simulink model "ADCS_orbiter_detumbling"  (R2022a)
settings: Solver=ode4  StartTime=0.0  StopTime=21085  FixedStep=0.1  MaxStep=1  RelTol=1e-8
values from neighbouring files (symbols this model uses):
  A_cube = 1    [Data_detumbling.m]    (also in main_orbiter_detumbling.m = 12.9)
  A_S2B = [1,0,0;0,-1,0;0,0,-1]    [Data_detumbling.m]
  alpha_x = deg2rad(6/3600)    [Data_detumbling.m]
  alpha_y = deg2rad(6/3600)    [Data_detumbling.m]
  alpha_z = deg2rad(40/3600)    [Data_detumbling.m]
  B_ast = pinv(B)    [Data_detumbling.m]
  ceps = cos(eps)    [Data_detumbling.m]    (also in main_orbiter_detumbling.m)
  F_max = 0.650    (= 0.65)    [Data_detumbling.m]    (also in main_orbiter_detumbling.m = 1.13)
  F_min = 0.160    (= 0.16)    [Data_detumbling.m]    (also in main_orbiter_detumbling.m = 0.19)
  J = [Jx,0,0 ... (first row only)    [Data_detumbling.m]    (also in DisturbanceEvaluation.m = {J_NSO; J_SO}; Thruster_sizing_2.m = diag([12043.36, 15990.19, 8547.84]); main_orbiter.m = J_SO; main_orbiter_detumbling.m = J_SO)
  k_dx = G*J(1,1)/max(diag(J))    [main_orbiter_detumbling.m]
  k_dy = G*J(2,2)/max(diag(J))    [main_orbiter_detumbling.m]
  k_dz = G*J(3,3)/max(diag(J))    [main_orbiter_detumbling.m]
  k_p = 0    [Data_detumbling.m]    (also in main_orbiter_detumbling.m)
  n1 = [1;0;0]    [Data_detumbling.m]    (also in main_orbiter_detumbling.m)
  n2 = [0;1;0]    [Data_detumbling.m]    (also in main_orbiter_detumbling.m)
  n3 = [0;0;1]    [Data_detumbling.m]    (also in main_orbiter_detumbling.m)
  n4 = -n1    [Data_detumbling.m]    (also in main_orbiter_detumbling.m)
  n5 = -n2    [Data_detumbling.m]    (also in main_orbiter_detumbling.m)
  n6 = -n3    [Data_detumbling.m]    (also in main_orbiter_detumbling.m)
  n_sun = 2*pi/(365.25*24*3600)    (= 1.99102127766e-07)    [Data_detumbling.m]    (also in main_orbiter_detumbling.m)
  P = F_e/c    [Data_detumbling.m]    (also in main_orbiter_detumbling.m)
  qbn0 = qrand./norm(qrand)    [main_orbiter.m]    (also in main_orbiter_detumbling.m)
  R = diag([lx_mb/2 ly_mb/2 lz_mb/2]) * [0  0  1  1  0  0 -1 -1 ... (first row only)    [Data_detumbling.m]    (also in main_orbiter_detumbling.m = 0.5*[-ly*cos(inc)              ly*cos(inc)            ly*cos)
  R_ast = pinv(R)    [Data_detumbling.m]    (also in main_orbiter_detumbling.m)
  r_i = r_cube * [n1,n2,n3,n4,n5,n6]    [Data_detumbling.m]    (also in main_orbiter_detumbling.m = [lx/2-cm_off_x  -cm_off_x       -cm_off_x        lx/2+cm_off)
  rho_d = 0.1    [Data_detumbling.m]    (also in main_orbiter_detumbling.m)
  rho_s = 0.5    [Data_detumbling.m]    (also in main_orbiter_detumbling.m)
  S_star1 = S_star1/norm(S_star1)    [Data_detumbling.m]
  S_star2 = S_star2/norm(S_star2)    [Data_detumbling.m]
  S_star3 = S_star3/norm(S_star3)    [Data_detumbling.m]
  S_star4 = S_star4/norm(S_star4)    [Data_detumbling.m]
  seps = sin(eps)    [Data_detumbling.m]    (also in main_orbiter_detumbling.m)
  sigma_ARW = deg2rad(0.001)    [main_orbiter_detumbling.m]
  state0 = [r_vec_new; v_vec_new]    [main_orbiter_detumbling.m]
  w = ones(length(R(1,:)),1)    [Data_detumbling.m]    (also in main_orbiter_detumbling.m)
  w_c = [0 0 0]'    [Data_detumbling.m]    (also in main_orbiter_detumbling.m)
  wb0 = 0.0001*rand(3, 1)    [main_orbiter.m]    (also in main_orbiter_detumbling.m = 0.1*rand(3, 1))
libraries: vrlib x8, matrix_library x1, simulink x1
(part 2 of 3)

== system ADCS_orbiter_detumbling/Actuators/Subsystem4/If Action Subsystem ==
  In1 : Inport
  Action Port : ActionPort  ActionPortLabel=if(u1 > F_max)
  Out1 : Outport
  wires:
  In1/1 -> Out1/1

== system ADCS_orbiter_detumbling/Actuators/Subsystem4/If Action Subsystem1 ==
  In1 : Inport
  Action Port : ActionPort  ActionPortLabel=elseif(u1<F_min)
  Out1 : Outport
  wires:
  In1/1 -> Out1/1

== system ADCS_orbiter_detumbling/Actuators/Subsystem4/If Action Subsystem2 ==
  In1 : Inport
  Action Port : ActionPort  ActionPortLabel=else
  Out1 : Outport
  wires:
  In1/1 -> Out1/1

== system ADCS_orbiter_detumbling/Actuators/Subsystem5/If Action Subsystem ==
  In1 : Inport
  Action Port : ActionPort  ActionPortLabel=if(u1 > F_max)
  Out1 : Outport
  wires:
  In1/1 -> Out1/1

== system ADCS_orbiter_detumbling/Actuators/Subsystem5/If Action Subsystem1 ==
  In1 : Inport
  Action Port : ActionPort  ActionPortLabel=elseif(u1<F_min)
  Out1 : Outport
  wires:
  In1/1 -> Out1/1

== system ADCS_orbiter_detumbling/Actuators/Subsystem5/If Action Subsystem2 ==
  In1 : Inport
  Action Port : ActionPort  ActionPortLabel=else
  Out1 : Outport
  wires:
  In1/1 -> Out1/1

== system ADCS_orbiter_detumbling/Actuators/Subsystem6/If Action Subsystem ==
  In1 : Inport
  Action Port : ActionPort  ActionPortLabel=if(u1 > F_max)
  Out1 : Outport
  wires:
  In1/1 -> Out1/1

== system ADCS_orbiter_detumbling/Actuators/Subsystem6/If Action Subsystem1 ==
  In1 : Inport
  Action Port : ActionPort  ActionPortLabel=elseif(u1<F_min)
  Out1 : Outport
  wires:
  In1/1 -> Out1/1

== system ADCS_orbiter_detumbling/Actuators/Subsystem6/If Action Subsystem2 ==
  In1 : Inport
  Action Port : ActionPort  ActionPortLabel=else
  Out1 : Outport
  wires:
  In1/1 -> Out1/1

== system ADCS_orbiter_detumbling/Actuators/Subsystem7/If Action Subsystem ==
  In1 : Inport
  Action Port : ActionPort  ActionPortLabel=if(u1 > F_max)
  Out1 : Outport
  wires:
  In1/1 -> Out1/1

== system ADCS_orbiter_detumbling/Actuators/Subsystem7/If Action Subsystem1 ==
  In1 : Inport
  Action Port : ActionPort  ActionPortLabel=elseif(u1<F_min)
  Out1 : Outport
  wires:
  In1/1 -> Out1/1

== system ADCS_orbiter_detumbling/Actuators/Subsystem7/If Action Subsystem2 ==
  In1 : Inport
  Action Port : ActionPort  ActionPortLabel=else
  Out1 : Outport
  wires:
  In1/1 -> Out1/1

== system ADCS_orbiter_detumbling/Actuators/Subsystem8/If Action Subsystem ==
  In1 : Inport
  Action Port : ActionPort  ActionPortLabel=if(u1 > 0)
  Out2 : Outport
  wires:
  In1/1 -> Out2/1

== system ADCS_orbiter_detumbling/Actuators/Subsystem8/If Action Subsystem1 ==
  In1 : Inport
  Input : Inport  Port=2
  Input1 : Inport  Port=3
  Action Port : ActionPort  ActionPortLabel=else
  If : If  NumInputs=2  IfExpression=u1 > 0 & u2==0
  If Action Subsystem : Subsystem  TreatAsAtomicUnit=on
  If Action Subsystem1 : Subsystem  TreatAsAtomicUnit=on
  Merge : Merge
  Out1 : Outport
  wires:
  In1/1 -> If Action Subsystem1/1(In1)
  Input/1 -> If/1  "u(k-1)"
  Input1/1 -> If/2  "u(k-2)"
  If/1 -> If Action Subsystem/Action
  If/2 -> If Action Subsystem1/Action
  If Action Subsystem1/1(Out1) -> Merge/2
  If Action Subsystem/1(Out1) -> Merge/1
  Merge/1 -> Out1/1

== system ADCS_orbiter_detumbling/Actuators/Subsystem9/If Action Subsystem ==
  In1 : Inport
  Action Port : ActionPort  ActionPortLabel=if(u1 > 0)
  Out2 : Outport
  wires:
  In1/1 -> Out2/1

== system ADCS_orbiter_detumbling/Actuators/Subsystem9/If Action Subsystem1 ==
  In1 : Inport
  Input : Inport  Port=2
  Input1 : Inport  Port=3
  Action Port : ActionPort  ActionPortLabel=else
  If : If  NumInputs=2  IfExpression=u1 > 0 & u2==0
  If Action Subsystem : Subsystem  TreatAsAtomicUnit=on
  If Action Subsystem1 : Subsystem  TreatAsAtomicUnit=on
  Merge : Merge
  Out1 : Outport
  wires:
  Merge/1 -> Out1/1
  If Action Subsystem/1(Out1) -> Merge/1
  If Action Subsystem1/1(Out1) -> Merge/2
  If/2 -> If Action Subsystem1/Action
  If/1 -> If Action Subsystem/Action
  Input1/1 -> If/2  "u(k-2)"
  Input/1 -> If/1  "u(k-1)"
  In1/1 -> If Action Subsystem1/1(In1)

== system ADCS_orbiter_detumbling/Control/target quaterion/Mapping choice ==
  A_I2B_target : Inport
  From q4 : Subsystem
  If Action Subsystem2 : Subsystem  TreatAsAtomicUnit=on
  If Action Subsystem3 : Subsystem  TreatAsAtomicUnit=on
  If1 : If  NumInputs=2  IfExpression=u1 == u2
  Max : MinMax  Function=max  Inputs=4
  Merge1 : Merge
  q_1 : Subsystem
  q_2 : Subsystem
  q_3 : Subsystem
  q_4 : Subsystem
  q_c : Outport
  wires:
  Merge1/1 -> q_c/1  "q_err"
  q_4/1(q4) -> Max/4, From q4/2(q4), If1/1  "q4"
  q_3/1(q3) -> Max/3, If Action Subsystem2/5(q3)  "q3"
  q_2/1(q2) -> Max/2, If Action Subsystem2/4(q2)  "q2"
  q_1/1(q1) -> Max/1, If Action Subsystem2/3(q1)  "q1"
  Max/1 -> If1/2, If Action Subsystem2/1(max)  "max"
  From q4/1(q_err) -> If Action Subsystem3/1(q_err)
  If Action Subsystem3/1("q_err from q4 ") -> Merge1/1
  A_I2B_target/1 -> If Action Subsystem2/2(A_I2B_err), q_1/1(A_I2B_err), q_2/1(A_I2B_err), From q4/1(A_I2B_err), q_4/1(A_I2B_err), q_3/1(A_I2B_err)
  If1/1 -> If Action Subsystem3/Action
  If1/2 -> If Action Subsystem2/Action
  If Action Subsystem2/1(Output) -> Merge1/2

== system ADCS_orbiter_detumbling/Environment 2/ShadowCylinder/If Action Subsystem ==
  Action Port : ActionPort  ActionPortLabel=if(u1 > 0)
  Constant : Constant
  Out1 : Outport
  wires:
  Constant/1 -> Out1/1

== system ADCS_orbiter_detumbling/Environment 2/ShadowCylinder/If Action Subsystem1 ==
  In1 : Inport
  Action Port : ActionPort  ActionPortLabel=else
  If : If
  If Action Subsystem : Subsystem  TreatAsAtomicUnit=on
  If Action Subsystem1 : Subsystem  TreatAsAtomicUnit=on
  Merge : Merge
  Out1 : Outport
  wires:
  In1/1 -> If/1
  If/1 -> If Action Subsystem/Action
  Merge/1 -> Out1/1
  If Action Subsystem/1(Out1) -> Merge/1
  If Action Subsystem1/1(Out1) -> Merge/2
  If/2 -> If Action Subsystem1/Action

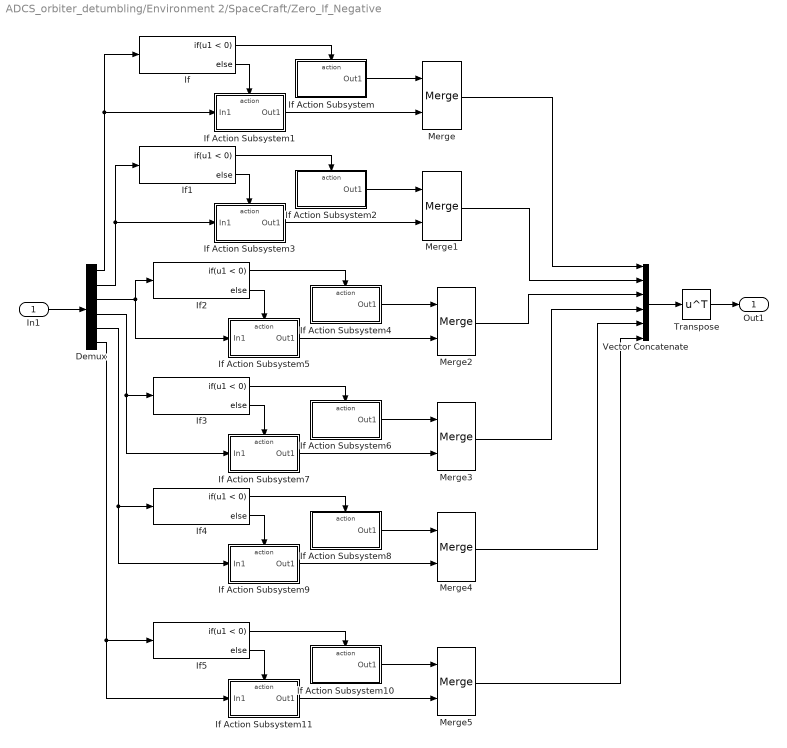
== system ADCS_orbiter_detumbling/Environment 2/SpaceCraft/Zero_If_Negative ==
  In1 : Inport
  Demux : Demux  Outputs=6
  If{,1..5} (6 alike) : If  IfExpression=u1 < 0
  If Action Subsystem : Subsystem  TreatAsAtomicUnit=on
  If Action Subsystem1 : Subsystem  TreatAsAtomicUnit=on
  If Action Subsystem10 : Subsystem  TreatAsAtomicUnit=on
  If Action Subsystem11 : Subsystem  TreatAsAtomicUnit=on
  If Action Subsystem2 : Subsystem  TreatAsAtomicUnit=on
  If Action Subsystem3 : Subsystem  TreatAsAtomicUnit=on
  If Action Subsystem4 : Subsystem  TreatAsAtomicUnit=on
  If Action Subsystem5 : Subsystem  TreatAsAtomicUnit=on
  If Action Subsystem6 : Subsystem  TreatAsAtomicUnit=on
  If Action Subsystem7 : Subsystem  TreatAsAtomicUnit=on
  If Action Subsystem8 : Subsystem  TreatAsAtomicUnit=on
  If Action Subsystem9 : Subsystem  TreatAsAtomicUnit=on
  Merge{,1..5} (6 alike) : Merge
  Transpose : Math  Operator=transpose
  Vector Concatenate : Concatenate  NumInputs=6
  Out1 : Outport
  wires:
  In1/1 -> Demux/1
  Vector Concatenate/1 -> Transpose/1
  Demux/1 -> If Action Subsystem1/1(In1), If/1
  If/1 -> If Action Subsystem/Action
  If Action Subsystem/1(Out1) -> Merge/1
  If Action Subsystem1/1(Out1) -> Merge/2
  If/2 -> If Action Subsystem1/Action
  If Action Subsystem2/1(Out1) -> Merge1/1
  Demux/2 -> If Action Subsystem3/1(In1), If1/1
  If1/1 -> If Action Subsystem2/Action
  If1/2 -> If Action Subsystem3/Action
  If Action Subsystem3/1(Out1) -> Merge1/2
  Merge/1 -> Vector Concatenate/1
  Merge1/1 -> Vector Concatenate/2
  If Action Subsystem4/1(Out1) -> Merge2/1
  Demux/3 -> If Action Subsystem5/1(In1), If2/1
  If2/1 -> If Action Subsystem4/Action
  If2/2 -> If Action Subsystem5/Action
  If Action Subsystem5/1(Out1) -> Merge2/2
  Merge2/1 -> Vector Concatenate/3
  If Action Subsystem6/1(Out1) -> Merge3/1
  Demux/4 -> If Action Subsystem7/1(In1), If3/1
  If3/1 -> If Action Subsystem6/Action
  If3/2 -> If Action Subsystem7/Action
  If Action Subsystem7/1(Out1) -> Merge3/2
  Merge3/1 -> Vector Concatenate/4
  If Action Subsystem8/1(Out1) -> Merge4/1
  Demux/5 -> If Action Subsystem9/1(In1), If4/1
  If4/1 -> If Action Subsystem8/Action
  If4/2 -> If Action Subsystem9/Action
  If Action Subsystem9/1(Out1) -> Merge4/2
  Merge4/1 -> Vector Concatenate/5
  If Action Subsystem10/1(Out1) -> Merge5/1
  Demux/6 -> If Action Subsystem11/1(In1), If5/1
  If5/1 -> If Action Subsystem10/Action
  If5/2 -> If Action Subsystem11/Action
  If Action Subsystem11/1(Out1) -> Merge5/2
  Merge5/1 -> Vector Concatenate/6
  Transpose/1 -> Out1/1

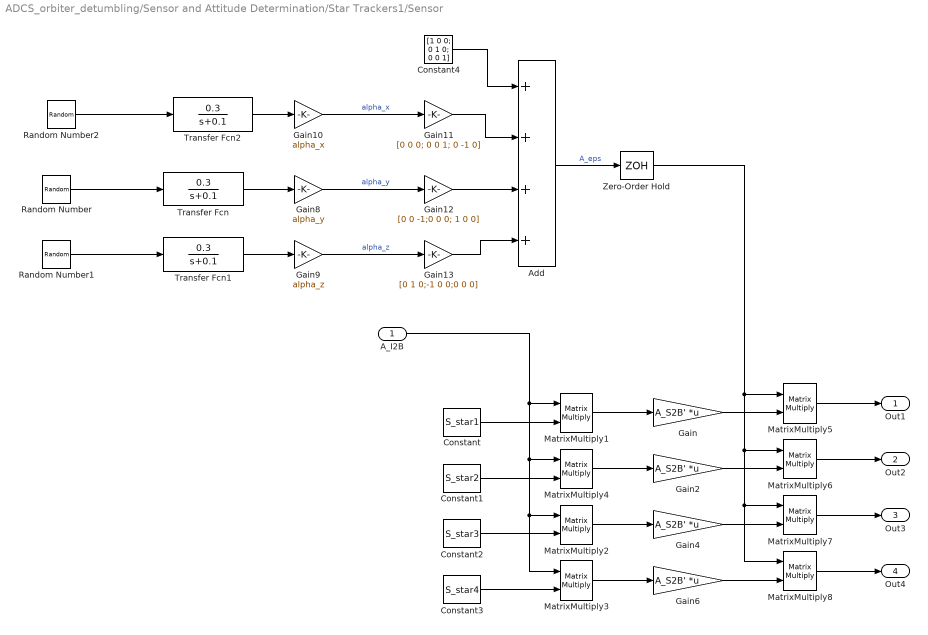
== system ADCS_orbiter_detumbling/Sensor and Attitude Determination/Star Trackers1/Sensor ==
  A_I2B : Inport
  Add : Sum  Inputs=++++
  Constant : Constant  Value=S_star1
  Constant1 : Constant  Value=S_star2
  Constant2 : Constant  Value=S_star3
  Constant3 : Constant  Value=S_star4
  Constant4 : Constant  Value=[1 0 0; 0 1 0; 0 0 1]
  Gain{,2,4,6} (4 alike) : Gain  Gain=A_S2B'  Multiplication=Matrix(K*u)
  Gain10 : Gain  Gain=alpha_x
  Gain11 : Gain  Gain=[0 0 0; 0 0 1; 0 -1 0]
  Gain12 : Gain  Gain=[0 0 -1;0 0 0; 1 0 0]
  Gain13 : Gain  Gain=[0 1 0;-1 0 0;0 0 0]
  Gain8 : Gain  Gain=alpha_y
  Gain9 : Gain  Gain=alpha_z
  MatrixMultiply{1..8} (8 alike) : Product  Multiplication=Matrix(*)
  Random Number : RandomNumber  SampleTime=0.1
  Random Number1 : RandomNumber  SampleTime=0.1
  Random Number2 : RandomNumber  SampleTime=0.1
  Transfer Fcn : TransferFcn  Numerator=[0.3]  Denominator=[1 0.1]
  Transfer Fcn1 : TransferFcn  Numerator=[0.3]  Denominator=[1 0.1]
  Transfer Fcn2 : TransferFcn  Numerator=[0.3]  Denominator=[1 0.1]
  Zero-Order Hold : ZeroOrderHold  SampleTime=-1
  Out1 : Outport
  Out2 : Outport  Port=2
  Out3 : Outport  Port=3
  Out4 : Outport  Port=4
  wires:
  MatrixMultiply1/1 -> Gain/1
  Constant/1 -> MatrixMultiply1/2
  A_I2B/1 -> MatrixMultiply3/1, MatrixMultiply2/1, MatrixMultiply4/1, MatrixMultiply1/1
  Constant1/1 -> MatrixMultiply4/2
  Gain6/1 -> MatrixMultiply8/2
  MatrixMultiply8/1 -> Out4/1
  Gain4/1 -> MatrixMultiply7/2
  MatrixMultiply6/1 -> Out2/1
  Constant3/1 -> MatrixMultiply3/2
  MatrixMultiply4/1 -> Gain2/1
  Constant2/1 -> MatrixMultiply2/2
  MatrixMultiply2/1 -> Gain4/1
  Gain2/1 -> MatrixMultiply6/2
  MatrixMultiply3/1 -> Gain6/1
  MatrixMultiply7/1 -> Out3/1
  MatrixMultiply5/1 -> Out1/1
  Gain9/1 -> Gain13/1  "alpha_z"
  Gain10/1 -> Gain11/1  "alpha_x"
  Transfer Fcn2/1 -> Gain10/1
  Random Number1/1 -> Transfer Fcn1/1
  Transfer Fcn1/1 -> Gain9/1
  Gain8/1 -> Gain12/1  "alpha_y"
  Random Number/1 -> Transfer Fcn/1
  Transfer Fcn/1 -> Gain8/1
  Random Number2/1 -> Transfer Fcn2/1
  Gain13/1 -> Add/4
  Gain12/1 -> Add/3
  Gain11/1 -> Add/2
  Constant4/1 -> Add/1
  Add/1 -> Zero-Order Hold/1  "A_eps"
  Gain/1 -> MatrixMultiply5/2
  Zero-Order Hold/1 -> MatrixMultiply5/1, MatrixMultiply6/1, MatrixMultiply7/1, MatrixMultiply8/1

== system ADCS_orbiter_detumbling/Sensor and Attitude Determination/Subsystem3/From q4 ==
  q4 : Inport
  A_I2B_err : Inport  Port=2
  Divide : Product  Inputs=*/
  Gain9 : Gain  Gain=4
  Selector3 : Selector  NumberOfDimensions=2  InputPortWidth=3  IndexOptions=Index vector (dialog),Index vector (dialog)  Indices=2,3  OutputSizes=1,1
  Selector4 : Selector  NumberOfDimensions=2  InputPortWidth=3  IndexOptions=Index vector (dialog),Index vector (dialog)  Indices=3,2  OutputSizes=1,1
  Selector5 : Selector  NumberOfDimensions=2  InputPortWidth=3  IndexOptions=Index vector (dialog),Index vector (dialog)  Indices=3,1  OutputSizes=1,1
  Selector6 : Selector  NumberOfDimensions=2  InputPortWidth=3  IndexOptions=Index vector (dialog),Index vector (dialog)  Indices=1,3  OutputSizes=1,1
  Selector7 : Selector  NumberOfDimensions=2  InputPortWidth=3  IndexOptions=Index vector (dialog),Index vector (dialog)  Indices=1,2  OutputSizes=1,1
  Selector8 : Selector  NumberOfDimensions=2  InputPortWidth=3  IndexOptions=Index vector (dialog),Index vector (dialog)  Indices=2,1  OutputSizes=1,1
  Sum1 : Sum  Inputs=+-
  Sum2 : Sum  Inputs=+-
  Sum3 : Sum  Inputs=+-
  Vector Concatenate : Concatenate
  Vector Concatenate2 : Concatenate  NumInputs=3
  q_err : Outport
  wires:
  Vector Concatenate2/1 -> Divide/1
  Selector7/1 -> Sum3/1
  Selector5/1 -> Sum2/1
  Divide/1 -> Vector Concatenate/1
  Selector3/1 -> Sum1/1
  Selector8/1 -> Sum3/2
  Sum2/1 -> Vector Concatenate2/2
  Vector Concatenate/1 -> q_err/1
  A_I2B_err/1 -> Selector3/1, Selector4/1, Selector5/1, Selector6/1, Selector7/1, Selector8/1
  Gain9/1 -> Divide/2
  Sum1/1 -> Vector Concatenate2/1
  q4/1 -> Gain9/1, Vector Concatenate/2  "q4"
  Selector4/1 -> Sum1/2
  Sum3/1 -> Vector Concatenate2/3
  Selector6/1 -> Sum2/2

== system ADCS_orbiter_detumbling/Sensor and Attitude Determination/Subsystem3/Mapping choice ==
  A_I2B_err1 : Inport
  From q4 : Subsystem
  If Action Subsystem2 : Subsystem  TreatAsAtomicUnit=on
  If Action Subsystem3 : Subsystem  TreatAsAtomicUnit=on
  If1 : If  NumInputs=2  IfExpression=u1 == u2
  Max : MinMax  Function=max  Inputs=4
  Merge1 : Merge
  q_1 : Subsystem
  q_2 : Subsystem
  q_3 : Subsystem
  q_4 : Subsystem
  q_err : Outport
  wires:
  Merge1/1 -> q_err/1  "q_err"
  q_4/1(q4) -> Max/4, From q4/2(q4), If1/1  "q4"
  q_3/1(q3) -> Max/3, If Action Subsystem2/5(q3)  "q3"
  q_2/1(q2) -> Max/2, If Action Subsystem2/4(q2)  "q2"
  q_1/1(q1) -> Max/1, If Action Subsystem2/3(q1)  "q1"
  Max/1 -> If1/2, If Action Subsystem2/1(max)  "max"
  From q4/1(q_err) -> If Action Subsystem3/1(q_err)
  If Action Subsystem3/1("q_err from q4 ") -> Merge1/1
  A_I2B_err1/1 -> If Action Subsystem2/2(A_I2B_err), q_1/1(A_I2B_err), q_2/1(A_I2B_err), From q4/1(A_I2B_err), q_4/1(A_I2B_err), q_3/1(A_I2B_err)
  If1/1 -> If Action Subsystem3/Action
  If1/2 -> If Action Subsystem2/Action
  If Action Subsystem2/1(Output) -> Merge1/2

== system ADCS_orbiter_detumbling/Actuators/Subsystem10/If Action Subsystem1/If Action Subsystem ==
  Action Port : ActionPort  ActionPortLabel=if(u1 > 0 & u2==0)
  Constant : Constant  Value=F_min
  Out1 : Outport
  wires:
  Constant/1 -> Out1/1

== system ADCS_orbiter_detumbling/Actuators/Subsystem10/If Action Subsystem1/If Action Subsystem1 ==
  In1 : Inport
  Action Port : ActionPort  ActionPortLabel=else
  Out1 : Outport
  wires:
  In1/1 -> Out1/1

== system ADCS_orbiter_detumbling/Actuators/Subsystem11/If Action Subsystem1/If Action Subsystem ==
  Action Port : ActionPort  ActionPortLabel=if(u1 > 0 & u2==0)
  Constant : Constant  Value=F_min
  Out1 : Outport
  wires:
  Constant/1 -> Out1/1

== system ADCS_orbiter_detumbling/Actuators/Subsystem11/If Action Subsystem1/If Action Subsystem1 ==
  In1 : Inport
  Action Port : ActionPort  ActionPortLabel=else
  Out1 : Outport
  wires:
  In1/1 -> Out1/1

== system ADCS_orbiter_detumbling/Actuators/Subsystem12/If Action Subsystem1/If Action Subsystem ==
  Action Port : ActionPort  ActionPortLabel=if(u1 > 0 & u2==0)
  Constant : Constant  Value=F_min
  Out1 : Outport
  wires:
  Constant/1 -> Out1/1

== system ADCS_orbiter_detumbling/Actuators/Subsystem12/If Action Subsystem1/If Action Subsystem1 ==
  In1 : Inport
  Action Port : ActionPort  ActionPortLabel=else
  Out1 : Outport
  wires:
  In1/1 -> Out1/1

== system ADCS_orbiter_detumbling/Actuators/Subsystem13/If Action Subsystem1/If Action Subsystem ==
  Action Port : ActionPort  ActionPortLabel=if(u1 > 0 & u2==0)
  Constant : Constant  Value=F_min
  Out1 : Outport
  wires:
  Constant/1 -> Out1/1

== system ADCS_orbiter_detumbling/Actuators/Subsystem13/If Action Subsystem1/If Action Subsystem1 ==
  In1 : Inport
  Action Port : ActionPort  ActionPortLabel=else
  Out1 : Outport
  wires:
  In1/1 -> Out1/1

== system ADCS_orbiter_detumbling/Actuators/Subsystem14/If Action Subsystem1/If Action Subsystem ==
  Action Port : ActionPort  ActionPortLabel=if(u1 > 0 & u2==0)
  Constant : Constant  Value=F_min
  Out1 : Outport
  wires:
  Constant/1 -> Out1/1

== system ADCS_orbiter_detumbling/Actuators/Subsystem14/If Action Subsystem1/If Action Subsystem1 ==
  In1 : Inport
  Action Port : ActionPort  ActionPortLabel=else
  Out1 : Outport
  wires:
  In1/1 -> Out1/1

== system ADCS_orbiter_detumbling/Actuators/Subsystem15/If Action Subsystem1/If Action Subsystem ==
  Action Port : ActionPort  ActionPortLabel=if(u1 > 0 & u2==0)
  Constant : Constant  Value=F_min
  Out1 : Outport
  wires:
  Constant/1 -> Out1/1

== system ADCS_orbiter_detumbling/Actuators/Subsystem15/If Action Subsystem1/If Action Subsystem1 ==
  In1 : Inport
  Action Port : ActionPort  ActionPortLabel=else
  Out1 : Outport
  wires:
  In1/1 -> Out1/1

== system ADCS_orbiter_detumbling/Actuators/Subsystem8/If Action Subsystem1/If Action Subsystem ==
  Action Port : ActionPort  ActionPortLabel=if(u1 > 0 & u2==0)
  Constant : Constant  Value=F_min
  Out1 : Outport
  wires:
  Constant/1 -> Out1/1

== system ADCS_orbiter_detumbling/Actuators/Subsystem8/If Action Subsystem1/If Action Subsystem1 ==
  In1 : Inport
  Action Port : ActionPort  ActionPortLabel=else
  Out1 : Outport
  wires:
  In1/1 -> Out1/1

== system ADCS_orbiter_detumbling/Actuators/Subsystem9/If Action Subsystem1/If Action Subsystem ==
  Action Port : ActionPort  ActionPortLabel=if(u1 > 0 & u2==0)
  Constant : Constant  Value=F_min
  Out1 : Outport
  wires:
  Constant/1 -> Out1/1

== system ADCS_orbiter_detumbling/Actuators/Subsystem9/If Action Subsystem1/If Action Subsystem1 ==
  In1 : Inport
  Action Port : ActionPort  ActionPortLabel=else
  Out1 : Outport
  wires:
  In1/1 -> Out1/1

== system ADCS_orbiter_detumbling/Control/target quaterion/Mapping choice/From q4 ==
  A_I2B_err : Inport
  q4 : Inport  Port=2
  Divide : Product  Inputs=*/
  Gain9 : Gain  Gain=4
  Selector3 : Selector  NumberOfDimensions=2  InputPortWidth=3  IndexOptions=Index vector (dialog),Index vector (dialog)  Indices=2,3  OutputSizes=1,1
  Selector4 : Selector  NumberOfDimensions=2  InputPortWidth=3  IndexOptions=Index vector (dialog),Index vector (dialog)  Indices=3,2  OutputSizes=1,1
  Selector5 : Selector  NumberOfDimensions=2  InputPortWidth=3  IndexOptions=Index vector (dialog),Index vector (dialog)  Indices=3,1  OutputSizes=1,1
  Selector6 : Selector  NumberOfDimensions=2  InputPortWidth=3  IndexOptions=Index vector (dialog),Index vector (dialog)  Indices=1,3  OutputSizes=1,1
  Selector7 : Selector  NumberOfDimensions=2  InputPortWidth=3  IndexOptions=Index vector (dialog),Index vector (dialog)  Indices=1,2  OutputSizes=1,1
  Selector8 : Selector  NumberOfDimensions=2  InputPortWidth=3  IndexOptions=Index vector (dialog),Index vector (dialog)  Indices=2,1  OutputSizes=1,1
  Sum1 : Sum  Inputs=+-
  Sum2 : Sum  Inputs=+-
  Sum3 : Sum  Inputs=+-
  Vector Concatenate : Concatenate
  Vector Concatenate2 : Concatenate  NumInputs=3
  q_err : Outport
  wires:
  Vector Concatenate2/1 -> Divide/1
  Selector7/1 -> Sum3/1
  Selector5/1 -> Sum2/1
  Divide/1 -> Vector Concatenate/1
  Selector3/1 -> Sum1/1
  Selector8/1 -> Sum3/2
  Sum2/1 -> Vector Concatenate2/2
  Vector Concatenate/1 -> q_err/1
  A_I2B_err/1 -> Selector3/1, Selector4/1, Selector5/1, Selector6/1, Selector7/1, Selector8/1
  Gain9/1 -> Divide/2
  Sum1/1 -> Vector Concatenate2/1
  q4/1 -> Gain9/1, Vector Concatenate/2  "q4"
  Selector4/1 -> Sum1/2
  Sum3/1 -> Vector Concatenate2/3
  Selector6/1 -> Sum2/2

== system ADCS_orbiter_detumbling/Control/target quaterion/Mapping choice/If Action Subsystem2 ==
  max : Inport
  A_I2B_err : Inport  Port=2
  q1 : Inport  Port=3
  q2 : Inport  Port=4
  q3 : Inport  Port=5
  Action Port : ActionPort  ActionPortLabel=else
  From q1 : Subsystem
  If : If  NumInputs=2  IfExpression=u1 == u2
  If Action Subsystem : Subsystem  TreatAsAtomicUnit=on
  If Action Subsystem1 : Subsystem  TreatAsAtomicUnit=on
  Merge : Merge
  Output : Outport
  wires:
  max/1 -> If/2, If Action Subsystem/1(max)
  Merge/1 -> Output/1
  If Action Subsystem/1(Output) -> Merge/2
  If Action Subsystem1/1(q_err from q1) -> Merge/1
  From q1/1(q_err) -> If Action Subsystem1/1(q_err)
  A_I2B_err/1 -> From q1/1(A_I2B_err), If Action Subsystem/2(A_I2B_err)
  If/1 -> If Action Subsystem1/Action
  q3/1 -> If Action Subsystem/4(q3)
  q2/1 -> If Action Subsystem/3(q2)
  If/2 -> If Action Subsystem/Action
  q1/1 -> If/1, From q1/2(q1)

== system ADCS_orbiter_detumbling/Control/target quaterion/Mapping choice/If Action Subsystem3 ==
  q_err : Inport
  Action Port : ActionPort  ActionPortLabel=if(u1 == u2)
  "q_err from q4 " : Outport
  wires:
  q_err/1 -> "q_err from q4 "/1

== system ADCS_orbiter_detumbling/Control/target quaterion/Mapping choice/q_1 ==
  A_I2B_err : Inport
  Constant5 : Constant
  Gain8 : Gain  Gain=1/2
  Selector : Selector  NumberOfDimensions=2  InputPortWidth=3  IndexOptions=Index vector (dialog),Index vector (dialog)  Indices=1,1  OutputSizes=1,1
  Selector1 : Selector  NumberOfDimensions=2  InputPortWidth=3  IndexOptions=Index vector (dialog),Index vector (dialog)  Indices=2,2  OutputSizes=1,1
  Selector2 : Selector  NumberOfDimensions=2  InputPortWidth=3  IndexOptions=Index vector (dialog),Index vector (dialog)  Indices=3,3  OutputSizes=1,1
  Sqrt : Sqrt
  Sum : Sum  Inputs=++--
  q1 : Outport
  wires:
  Constant5/1 -> Sum/1
  Sum/1 -> Sqrt/1
  A_I2B_err/1 -> Selector1/1, Selector2/1, Selector/1
  Sqrt/1 -> Gain8/1
  Selector1/1 -> Sum/3
  Selector/1 -> Sum/2
  Selector2/1 -> Sum/4
  Gain8/1 -> q1/1  "q1"

== system ADCS_orbiter_detumbling/Control/target quaterion/Mapping choice/q_2 ==
  A_I2B_err : Inport
  Constant5 : Constant
  Gain8 : Gain  Gain=1/2
  Selector : Selector  NumberOfDimensions=2  InputPortWidth=3  IndexOptions=Index vector (dialog),Index vector (dialog)  Indices=1,1  OutputSizes=1,1
  Selector1 : Selector  NumberOfDimensions=2  InputPortWidth=3  IndexOptions=Index vector (dialog),Index vector (dialog)  Indices=2,2  OutputSizes=1,1
  Selector2 : Selector  NumberOfDimensions=2  InputPortWidth=3  IndexOptions=Index vector (dialog),Index vector (dialog)  Indices=3,3  OutputSizes=1,1
  Sqrt : Sqrt
  Sum : Sum  Inputs=+-+-
  q2 : Outport
  wires:
  Constant5/1 -> Sum/1
  Sum/1 -> Sqrt/1
  A_I2B_err/1 -> Selector1/1, Selector2/1, Selector/1
  Sqrt/1 -> Gain8/1
  Selector1/1 -> Sum/3
  Selector/1 -> Sum/2
  Selector2/1 -> Sum/4
  Gain8/1 -> q2/1  "q2"

== system ADCS_orbiter_detumbling/Control/target quaterion/Mapping choice/q_3 ==
  A_I2B_err : Inport
  Constant5 : Constant
  Gain8 : Gain  Gain=1/2
  Selector : Selector  NumberOfDimensions=2  InputPortWidth=3  IndexOptions=Index vector (dialog),Index vector (dialog)  Indices=1,1  OutputSizes=1,1
  Selector1 : Selector  NumberOfDimensions=2  InputPortWidth=3  IndexOptions=Index vector (dialog),Index vector (dialog)  Indices=2,2  OutputSizes=1,1
  Selector2 : Selector  NumberOfDimensions=2  InputPortWidth=3  IndexOptions=Index vector (dialog),Index vector (dialog)  Indices=3,3  OutputSizes=1,1
  Sqrt : Sqrt
  Sum : Sum  Inputs=+--+
  q3 : Outport
  wires:
  Constant5/1 -> Sum/1
  Sum/1 -> Sqrt/1
  A_I2B_err/1 -> Selector1/1, Selector2/1, Selector/1
  Sqrt/1 -> Gain8/1
  Selector1/1 -> Sum/3
  Selector/1 -> Sum/2
  Selector2/1 -> Sum/4
  Gain8/1 -> q3/1  "q3"

== system ADCS_orbiter_detumbling/Control/target quaterion/Mapping choice/q_4 ==
  A_I2B_err : Inport
  Constant5 : Constant
  Gain8 : Gain  Gain=1/2
  Selector : Selector  NumberOfDimensions=2  InputPortWidth=3  IndexOptions=Index vector (dialog),Index vector (dialog)  Indices=1,1  OutputSizes=1,1
  Selector1 : Selector  NumberOfDimensions=2  InputPortWidth=3  IndexOptions=Index vector (dialog),Index vector (dialog)  Indices=2,2  OutputSizes=1,1
  Selector2 : Selector  NumberOfDimensions=2  InputPortWidth=3  IndexOptions=Index vector (dialog),Index vector (dialog)  Indices=3,3  OutputSizes=1,1
  Sqrt : Sqrt
  Sum : Sum  Inputs=++++
  q4 : Outport
  wires:
  Constant5/1 -> Sum/1
  Sum/1 -> Sqrt/1
  A_I2B_err/1 -> Selector1/1, Selector2/1, Selector/1
  Sqrt/1 -> Gain8/1
  Selector1/1 -> Sum/3
  Selector/1 -> Sum/2
  Selector2/1 -> Sum/4
  Gain8/1 -> q4/1  "q4"

== system ADCS_orbiter_detumbling/Environment 2/ShadowCylinder/If Action Subsystem1/If Action Subsystem ==
  Action Port : ActionPort  ActionPortLabel=if(u1 > 0)
  Constant : Constant  Value=0
  Out1 : Outport
  wires:
  Constant/1 -> Out1/1

== system ADCS_orbiter_detumbling/Environment 2/ShadowCylinder/If Action Subsystem1/If Action Subsystem1 ==
  Action Port : ActionPort  ActionPortLabel=else
  Constant : Constant
  Out1 : Outport
  wires:
  Constant/1 -> Out1/1

== system ADCS_orbiter_detumbling/Environment 2/SpaceCraft/Zero_If_Negative/If Action Subsystem ==
  Action Port : ActionPort  ActionPortLabel=if(u1 < 0)
  Constant : Constant  Value=0
  Out1 : Outport
  wires:
  Constant/1 -> Out1/1

== system ADCS_orbiter_detumbling/Environment 2/SpaceCraft/Zero_If_Negative/If Action Subsystem1 ==
  In1 : Inport
  Action Port : ActionPort  ActionPortLabel=else
  Out1 : Outport
  wires:
  In1/1 -> Out1/1

== system ADCS_orbiter_detumbling/Environment 2/SpaceCraft/Zero_If_Negative/If Action Subsystem10 ==
  Action Port : ActionPort  ActionPortLabel=if(u1 < 0)
  Constant : Constant  Value=0
  Out1 : Outport
  wires:
  Constant/1 -> Out1/1

== system ADCS_orbiter_detumbling/Environment 2/SpaceCraft/Zero_If_Negative/If Action Subsystem11 ==
  In1 : Inport
  Action Port : ActionPort  ActionPortLabel=else
  Out1 : Outport
  wires:
  In1/1 -> Out1/1

== system ADCS_orbiter_detumbling/Environment 2/SpaceCraft/Zero_If_Negative/If Action Subsystem2 ==
  Action Port : ActionPort  ActionPortLabel=if(u1 < 0)
  Constant : Constant  Value=0
  Out1 : Outport
  wires:
  Constant/1 -> Out1/1

== system ADCS_orbiter_detumbling/Environment 2/SpaceCraft/Zero_If_Negative/If Action Subsystem3 ==
  In1 : Inport
  Action Port : ActionPort  ActionPortLabel=else
  Out1 : Outport
  wires:
  In1/1 -> Out1/1

== system ADCS_orbiter_detumbling/Environment 2/SpaceCraft/Zero_If_Negative/If Action Subsystem4 ==
  Action Port : ActionPort  ActionPortLabel=if(u1 < 0)
  Constant : Constant  Value=0
  Out1 : Outport
  wires:
  Constant/1 -> Out1/1

== system ADCS_orbiter_detumbling/Environment 2/SpaceCraft/Zero_If_Negative/If Action Subsystem5 ==
  In1 : Inport
  Action Port : ActionPort  ActionPortLabel=else
  Out1 : Outport
  wires:
  In1/1 -> Out1/1

== system ADCS_orbiter_detumbling/Environment 2/SpaceCraft/Zero_If_Negative/If Action Subsystem6 ==
  Action Port : ActionPort  ActionPortLabel=if(u1 < 0)
  Constant : Constant  Value=0
  Out1 : Outport
  wires:
  Constant/1 -> Out1/1

== system ADCS_orbiter_detumbling/Environment 2/SpaceCraft/Zero_If_Negative/If Action Subsystem7 ==
  In1 : Inport
  Action Port : ActionPort  ActionPortLabel=else
  Out1 : Outport
  wires:
  In1/1 -> Out1/1

== system ADCS_orbiter_detumbling/Environment 2/SpaceCraft/Zero_If_Negative/If Action Subsystem8 ==
  Action Port : ActionPort  ActionPortLabel=if(u1 < 0)
  Constant : Constant  Value=0
  Out1 : Outport
  wires:
  Constant/1 -> Out1/1

== system ADCS_orbiter_detumbling/Environment 2/SpaceCraft/Zero_If_Negative/If Action Subsystem9 ==
  In1 : Inport
  Action Port : ActionPort  ActionPortLabel=else
  Out1 : Outport
  wires:
  In1/1 -> Out1/1

== system ADCS_orbiter_detumbling/Sensor and Attitude Determination/Subsystem3/Mapping choice/From q4 ==
  A_I2B_err : Inport
  q4 : Inport  Port=2
  Divide : Product  Inputs=*/
  Gain9 : Gain  Gain=4
  Selector3 : Selector  NumberOfDimensions=2  InputPortWidth=3  IndexOptions=Index vector (dialog),Index vector (dialog)  Indices=2,3  OutputSizes=1,1
  Selector4 : Selector  NumberOfDimensions=2  InputPortWidth=3  IndexOptions=Index vector (dialog),Index vector (dialog)  Indices=3,2  OutputSizes=1,1
  Selector5 : Selector  NumberOfDimensions=2  InputPortWidth=3  IndexOptions=Index vector (dialog),Index vector (dialog)  Indices=3,1  OutputSizes=1,1
  Selector6 : Selector  NumberOfDimensions=2  InputPortWidth=3  IndexOptions=Index vector (dialog),Index vector (dialog)  Indices=1,3  OutputSizes=1,1
  Selector7 : Selector  NumberOfDimensions=2  InputPortWidth=3  IndexOptions=Index vector (dialog),Index vector (dialog)  Indices=1,2  OutputSizes=1,1
  Selector8 : Selector  NumberOfDimensions=2  InputPortWidth=3  IndexOptions=Index vector (dialog),Index vector (dialog)  Indices=2,1  OutputSizes=1,1
  Sum1 : Sum  Inputs=+-
  Sum2 : Sum  Inputs=+-
  Sum3 : Sum  Inputs=+-
  Vector Concatenate : Concatenate
  Vector Concatenate2 : Concatenate  NumInputs=3
  q_err : Outport
  wires:
  Vector Concatenate2/1 -> Divide/1
  Selector7/1 -> Sum3/1
  Selector5/1 -> Sum2/1
  Divide/1 -> Vector Concatenate/1
  Selector3/1 -> Sum1/1
  Selector8/1 -> Sum3/2
  Sum2/1 -> Vector Concatenate2/2
  Vector Concatenate/1 -> q_err/1
  A_I2B_err/1 -> Selector3/1, Selector4/1, Selector5/1, Selector6/1, Selector7/1, Selector8/1
  Gain9/1 -> Divide/2
  Sum1/1 -> Vector Concatenate2/1
  q4/1 -> Gain9/1, Vector Concatenate/2  "q4"
  Selector4/1 -> Sum1/2
  Sum3/1 -> Vector Concatenate2/3
  Selector6/1 -> Sum2/2

== system ADCS_orbiter_detumbling/Sensor and Attitude Determination/Subsystem3/Mapping choice/If Action Subsystem2 ==
  max : Inport
  A_I2B_err : Inport  Port=2
  q1 : Inport  Port=3
  q2 : Inport  Port=4
  q3 : Inport  Port=5
  Action Port : ActionPort  ActionPortLabel=else
  From q1 : Subsystem
  If : If  NumInputs=2  IfExpression=u1 == u2
  If Action Subsystem : Subsystem  TreatAsAtomicUnit=on
  If Action Subsystem1 : Subsystem  TreatAsAtomicUnit=on
  Merge : Merge
  Output : Outport
  wires:
  max/1 -> If/2, If Action Subsystem/1(max)
  Merge/1 -> Output/1
  If Action Subsystem/1(Output) -> Merge/2
  If Action Subsystem1/1(q_err from q1) -> Merge/1
  From q1/1(q_err) -> If Action Subsystem1/1(q_err)
  A_I2B_err/1 -> From q1/1(A_I2B_err), If Action Subsystem/2(A_I2B_err)
  If/1 -> If Action Subsystem1/Action
  q3/1 -> If Action Subsystem/4(q3)
  q2/1 -> If Action Subsystem/3(q2)
  If/2 -> If Action Subsystem/Action
  q1/1 -> If/1, From q1/2(q1)

== system ADCS_orbiter_detumbling/Sensor and Attitude Determination/Subsystem3/Mapping choice/If Action Subsystem3 ==
  q_err : Inport
  Action Port : ActionPort  ActionPortLabel=if(u1 == u2)
  "q_err from q4 " : Outport
  wires:
  q_err/1 -> "q_err from q4 "/1

== system ADCS_orbiter_detumbling/Sensor and Attitude Determination/Subsystem3/Mapping choice/q_1 ==
  A_I2B_err : Inport
  Constant5 : Constant
  Gain8 : Gain  Gain=1/2
  Selector : Selector  NumberOfDimensions=2  InputPortWidth=3  IndexOptions=Index vector (dialog),Index vector (dialog)  Indices=1,1  OutputSizes=1,1
  Selector1 : Selector  NumberOfDimensions=2  InputPortWidth=3  IndexOptions=Index vector (dialog),Index vector (dialog)  Indices=2,2  OutputSizes=1,1
  Selector2 : Selector  NumberOfDimensions=2  InputPortWidth=3  IndexOptions=Index vector (dialog),Index vector (dialog)  Indices=3,3  OutputSizes=1,1
  Sqrt : Sqrt
  Sum : Sum  Inputs=++--
  q1 : Outport
  wires:
  Constant5/1 -> Sum/1
  Sum/1 -> Sqrt/1
  A_I2B_err/1 -> Selector1/1, Selector2/1, Selector/1
  Sqrt/1 -> Gain8/1
  Selector1/1 -> Sum/3
  Selector/1 -> Sum/2
  Selector2/1 -> Sum/4
  Gain8/1 -> q1/1  "q1"

== system ADCS_orbiter_detumbling/Sensor and Attitude Determination/Subsystem3/Mapping choice/q_2 ==
  A_I2B_err : Inport
  Constant5 : Constant
  Gain8 : Gain  Gain=1/2
  Selector : Selector  NumberOfDimensions=2  InputPortWidth=3  IndexOptions=Index vector (dialog),Index vector (dialog)  Indices=1,1  OutputSizes=1,1
  Selector1 : Selector  NumberOfDimensions=2  InputPortWidth=3  IndexOptions=Index vector (dialog),Index vector (dialog)  Indices=2,2  OutputSizes=1,1
  Selector2 : Selector  NumberOfDimensions=2  InputPortWidth=3  IndexOptions=Index vector (dialog),Index vector (dialog)  Indices=3,3  OutputSizes=1,1
  Sqrt : Sqrt
  Sum : Sum  Inputs=+-+-
  q2 : Outport
  wires:
  Constant5/1 -> Sum/1
  Sum/1 -> Sqrt/1
  A_I2B_err/1 -> Selector1/1, Selector2/1, Selector/1
  Sqrt/1 -> Gain8/1
  Selector1/1 -> Sum/3
  Selector/1 -> Sum/2
  Selector2/1 -> Sum/4
  Gain8/1 -> q2/1  "q2"

== system ADCS_orbiter_detumbling/Sensor and Attitude Determination/Subsystem3/Mapping choice/q_3 ==
  A_I2B_err : Inport
  Constant5 : Constant
  Gain8 : Gain  Gain=1/2
  Selector : Selector  NumberOfDimensions=2  InputPortWidth=3  IndexOptions=Index vector (dialog),Index vector (dialog)  Indices=1,1  OutputSizes=1,1
  Selector1 : Selector  NumberOfDimensions=2  InputPortWidth=3  IndexOptions=Index vector (dialog),Index vector (dialog)  Indices=2,2  OutputSizes=1,1
  Selector2 : Selector  NumberOfDimensions=2  InputPortWidth=3  IndexOptions=Index vector (dialog),Index vector (dialog)  Indices=3,3  OutputSizes=1,1
  Sqrt : Sqrt
  Sum : Sum  Inputs=+--+
  q3 : Outport
  wires:
  Constant5/1 -> Sum/1
  Sum/1 -> Sqrt/1
  A_I2B_err/1 -> Selector1/1, Selector2/1, Selector/1
  Sqrt/1 -> Gain8/1
  Selector1/1 -> Sum/3
  Selector/1 -> Sum/2
  Selector2/1 -> Sum/4
  Gain8/1 -> q3/1  "q3"

== system ADCS_orbiter_detumbling/Sensor and Attitude Determination/Subsystem3/Mapping choice/q_4 ==
  A_I2B_err : Inport
  Constant5 : Constant
  Gain8 : Gain  Gain=1/2
  Selector : Selector  NumberOfDimensions=2  InputPortWidth=3  IndexOptions=Index vector (dialog),Index vector (dialog)  Indices=1,1  OutputSizes=1,1
  Selector1 : Selector  NumberOfDimensions=2  InputPortWidth=3  IndexOptions=Index vector (dialog),Index vector (dialog)  Indices=2,2  OutputSizes=1,1
  Selector2 : Selector  NumberOfDimensions=2  InputPortWidth=3  IndexOptions=Index vector (dialog),Index vector (dialog)  Indices=3,3  OutputSizes=1,1
  Sqrt : Sqrt
  Sum : Sum  Inputs=++++
  q4 : Outport
  wires:
  Constant5/1 -> Sum/1
  Sum/1 -> Sqrt/1
  A_I2B_err/1 -> Selector1/1, Selector2/1, Selector/1
  Sqrt/1 -> Gain8/1
  Selector1/1 -> Sum/3
  Selector/1 -> Sum/2
  Selector2/1 -> Sum/4
  Gain8/1 -> q4/1  "q4"

== system ADCS_orbiter_detumbling/Control/target quaterion/Mapping choice/If Action Subsystem2/From q1 ==
  A_I2B_err : Inport
  q1 : Inport  Port=2
  Divide : Product  Inputs=*/
  Gain9 : Gain  Gain=4
  Selector3 : Selector  NumberOfDimensions=2  InputPortWidth=3  IndexOptions=Index vector (dialog),Index vector (dialog)  Indices=1,2  OutputSizes=1,1
  Selector4 : Selector  NumberOfDimensions=2  InputPortWidth=3  IndexOptions=Index vector (dialog),Index vector (dialog)  Indices=2,1  OutputSizes=1,1
  Selector5 : Selector  NumberOfDimensions=2  InputPortWidth=3  IndexOptions=Index vector (dialog),Index vector (dialog)  Indices=3,1  OutputSizes=1,1
  Selector6 : Selector  NumberOfDimensions=2  InputPortWidth=3  IndexOptions=Index vector (dialog),Index vector (dialog)  Indices=1,3  OutputSizes=1,1
  Selector7 : Selector  NumberOfDimensions=2  InputPortWidth=3  IndexOptions=Index vector (dialog),Index vector (dialog)  Indices=2,3  OutputSizes=1,1
  Selector8 : Selector  NumberOfDimensions=2  InputPortWidth=3  IndexOptions=Index vector (dialog),Index vector (dialog)  Indices=3,2  OutputSizes=1,1
  Sum1 : Sum
  Sum2 : Sum
  Sum3 : Sum  Inputs=+-
  Vector Concatenate : Concatenate
  Vector Concatenate2 : Concatenate  NumInputs=3
  q_err : Outport
  wires:
  Vector Concatenate2/1 -> Divide/1
  Selector7/1 -> Sum3/1
  Selector5/1 -> Sum2/1
  Divide/1 -> Vector Concatenate/2
  Selector3/1 -> Sum1/1
  Selector8/1 -> Sum3/2
  Sum2/1 -> Vector Concatenate2/2  "q3"
  Vector Concatenate/1 -> q_err/1
  A_I2B_err/1 -> Selector5/1, Selector6/1, Selector7/1, Selector8/1, Selector3/1, Selector4/1
  Gain9/1 -> Divide/2
  Sum1/1 -> Vector Concatenate2/1  "q2"
  q1/1 -> Gain9/1, Vector Concatenate/1  "q1"
  Selector4/1 -> Sum1/2
  Sum3/1 -> Vector Concatenate2/3  "q4"
  Selector6/1 -> Sum2/2

== system ADCS_orbiter_detumbling/Control/target quaterion/Mapping choice/If Action Subsystem2/If Action Subsystem ==
  max : Inport
  A_I2B_err : Inport  Port=2
  q2 : Inport  Port=3
  q3 : Inport  Port=4
  Action Port : ActionPort  ActionPortLabel=else
  From q2 : Subsystem
  If : If  NumInputs=2  IfExpression=u1 == u2
  If Action Subsystem : Subsystem  TreatAsAtomicUnit=on
  If Action Subsystem1 : Subsystem  TreatAsAtomicUnit=on
  Merge : Merge
  Output : Outport
  wires:
  Merge/1 -> Output/1
  max/1 -> If/2
  If Action Subsystem1/1(q_err from q3) -> Merge/2
  If Action Subsystem/1(q_err from q2) -> Merge/1
  From q2/1(q_err) -> If Action Subsystem/1(q_err)
  A_I2B_err/1 -> From q2/1(A_I2B_err), If Action Subsystem1/1(A_I2B_err)
  q3/1 -> If Action Subsystem1/2(q3)
  If/2 -> If Action Subsystem1/Action
  If/1 -> If Action Subsystem/Action
  q2/1 -> If/1, From q2/2(q2)

== system ADCS_orbiter_detumbling/Control/target quaterion/Mapping choice/If Action Subsystem2/If Action Subsystem1 ==
  q_err : Inport
  Action Port : ActionPort  ActionPortLabel=if(u1 == u2)
  q_err from q1 : Outport
  wires:
  q_err/1 -> q_err from q1/1

== system ADCS_orbiter_detumbling/Sensor and Attitude Determination/Subsystem3/Mapping choice/If Action Subsystem2/From q1 ==
  A_I2B_err : Inport
  q1 : Inport  Port=2
  Divide : Product  Inputs=*/
  Gain9 : Gain  Gain=4
  Selector3 : Selector  NumberOfDimensions=2  InputPortWidth=3  IndexOptions=Index vector (dialog),Index vector (dialog)  Indices=1,2  OutputSizes=1,1
  Selector4 : Selector  NumberOfDimensions=2  InputPortWidth=3  IndexOptions=Index vector (dialog),Index vector (dialog)  Indices=2,1  OutputSizes=1,1
  Selector5 : Selector  NumberOfDimensions=2  InputPortWidth=3  IndexOptions=Index vector (dialog),Index vector (dialog)  Indices=3,1  OutputSizes=1,1
  Selector6 : Selector  NumberOfDimensions=2  InputPortWidth=3  IndexOptions=Index vector (dialog),Index vector (dialog)  Indices=1,3  OutputSizes=1,1
  Selector7 : Selector  NumberOfDimensions=2  InputPortWidth=3  IndexOptions=Index vector (dialog),Index vector (dialog)  Indices=2,3  OutputSizes=1,1
  Selector8 : Selector  NumberOfDimensions=2  InputPortWidth=3  IndexOptions=Index vector (dialog),Index vector (dialog)  Indices=3,2  OutputSizes=1,1
  Sum1 : Sum
  Sum2 : Sum
  Sum3 : Sum  Inputs=+-
  Vector Concatenate : Concatenate
  Vector Concatenate2 : Concatenate  NumInputs=3
  q_err : Outport
  wires:
  Vector Concatenate2/1 -> Divide/1
  Selector7/1 -> Sum3/1
  Selector5/1 -> Sum2/1
  Divide/1 -> Vector Concatenate/2
  Selector3/1 -> Sum1/1
  Selector8/1 -> Sum3/2
  Sum2/1 -> Vector Concatenate2/2  "q3"
  Vector Concatenate/1 -> q_err/1
  A_I2B_err/1 -> Selector5/1, Selector6/1, Selector7/1, Selector8/1, Selector3/1, Selector4/1
  Gain9/1 -> Divide/2
  Sum1/1 -> Vector Concatenate2/1  "q2"
  q1/1 -> Gain9/1, Vector Concatenate/1  "q1"
  Selector4/1 -> Sum1/2
  Sum3/1 -> Vector Concatenate2/3  "q4"
  Selector6/1 -> Sum2/2

== system ADCS_orbiter_detumbling/Sensor and Attitude Determination/Subsystem3/Mapping choice/If Action Subsystem2/If Action Subsystem ==
  max : Inport
  A_I2B_err : Inport  Port=2
  q2 : Inport  Port=3
  q3 : Inport  Port=4
  Action Port : ActionPort  ActionPortLabel=else
  From q2 : Subsystem
  If : If  NumInputs=2  IfExpression=u1 == u2
  If Action Subsystem : Subsystem  TreatAsAtomicUnit=on
  If Action Subsystem1 : Subsystem  TreatAsAtomicUnit=on
  Merge : Merge
  Output : Outport
  wires:
  Merge/1 -> Output/1
  max/1 -> If/2
  If Action Subsystem1/1(q_err from q3) -> Merge/2
  If Action Subsystem/1(q_err from q2) -> Merge/1
  From q2/1(q_err) -> If Action Subsystem/1(q_err)
  A_I2B_err/1 -> From q2/1(A_I2B_err), If Action Subsystem1/1(A_I2B_err)
  q3/1 -> If Action Subsystem1/2(q3)
  If/2 -> If Action Subsystem1/Action
  If/1 -> If Action Subsystem/Action
  q2/1 -> If/1, From q2/2(q2)

== system ADCS_orbiter_detumbling/Sensor and Attitude Determination/Subsystem3/Mapping choice/If Action Subsystem2/If Action Subsystem1 ==
  q_err : Inport
  Action Port : ActionPort  ActionPortLabel=if(u1 == u2)
  q_err from q1 : Outport
  wires:
  q_err/1 -> q_err from q1/1

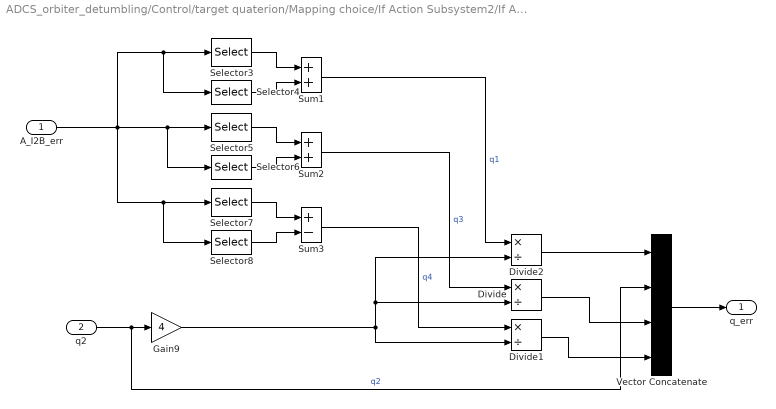
== system ADCS_orbiter_detumbling/Control/target quaterion/Mapping choice/If Action Subsystem2/If Action Subsystem/From q2 ==
  A_I2B_err : Inport
  q2 : Inport  Port=2
  Divide : Product  Inputs=*/
  Divide1 : Product  Inputs=*/
  Divide2 : Product  Inputs=*/
  Gain9 : Gain  Gain=4
  Selector3 : Selector  NumberOfDimensions=2  InputPortWidth=3  IndexOptions=Index vector (dialog),Index vector (dialog)  Indices=1,2  OutputSizes=1,1
  Selector4 : Selector  NumberOfDimensions=2  InputPortWidth=3  IndexOptions=Index vector (dialog),Index vector (dialog)  Indices=2,1  OutputSizes=1,1
  Selector5 : Selector  NumberOfDimensions=2  InputPortWidth=3  IndexOptions=Index vector (dialog),Index vector (dialog)  Indices=2,3  OutputSizes=1,1
  Selector6 : Selector  NumberOfDimensions=2  InputPortWidth=3  IndexOptions=Index vector (dialog),Index vector (dialog)  Indices=3,2  OutputSizes=1,1
  Selector7 : Selector  NumberOfDimensions=2  InputPortWidth=3  IndexOptions=Index vector (dialog),Index vector (dialog)  Indices=3,1  OutputSizes=1,1
  Selector8 : Selector  NumberOfDimensions=2  InputPortWidth=3  IndexOptions=Index vector (dialog),Index vector (dialog)  Indices=1,3  OutputSizes=1,1
  Sum1 : Sum
  Sum2 : Sum
  Sum3 : Sum  Inputs=+-
  Vector Concatenate : Concatenate  NumInputs=4
  q_err : Outport
  wires:
  Divide1/1 -> Vector Concatenate/4
  Divide/1 -> Vector Concatenate/3
  Divide2/1 -> Vector Concatenate/1
  Sum2/1 -> Divide/1  "q3"
  Selector7/1 -> Sum3/1
  Selector5/1 -> Sum2/1
  Selector3/1 -> Sum1/1
  Selector8/1 -> Sum3/2
  Vector Concatenate/1 -> q_err/1
  A_I2B_err/1 -> Selector5/1, Selector6/1, Selector7/1, Selector8/1, Selector3/1, Selector4/1
  Gain9/1 -> Divide2/2, Divide/2, Divide1/2
  Sum1/1 -> Divide2/1  "q1"
  q2/1 -> Gain9/1, Vector Concatenate/2  "q2"
  Selector4/1 -> Sum1/2
  Sum3/1 -> Divide1/1  "q4"
  Selector6/1 -> Sum2/2

== system ADCS_orbiter_detumbling/Control/target quaterion/Mapping choice/If Action Subsystem2/If Action Subsystem/If Action Subsystem ==
  q_err : Inport
  Action Port : ActionPort  ActionPortLabel=if(u1 == u2)
  q_err from q2 : Outport
  wires:
  q_err/1 -> q_err from q2/1

== system ADCS_orbiter_detumbling/Control/target quaterion/Mapping choice/If Action Subsystem2/If Action Subsystem/If Action Subsystem1 ==
  A_I2B_err : Inport
  q3 : Inport  Port=2
  Action Port : ActionPort  ActionPortLabel=else
  From q3 : Subsystem
  q_err from q3 : Outport
  wires:
  From q3/1(q_err) -> q_err from q3/1
  A_I2B_err/1 -> From q3/1(A_I2B_err)
  q3/1 -> From q3/2(q3)

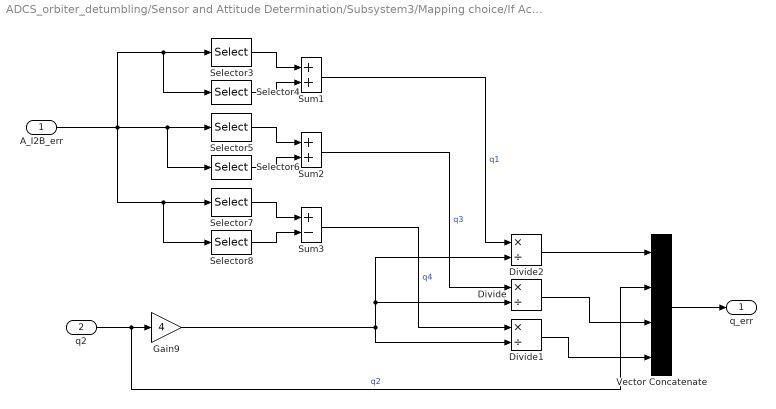
== system ADCS_orbiter_detumbling/Sensor and Attitude Determination/Subsystem3/Mapping choice/If Action Subsystem2/If Action Subsystem/From q2 ==
  A_I2B_err : Inport
  q2 : Inport  Port=2
  Divide : Product  Inputs=*/
  Divide1 : Product  Inputs=*/
  Divide2 : Product  Inputs=*/
  Gain9 : Gain  Gain=4
  Selector3 : Selector  NumberOfDimensions=2  InputPortWidth=3  IndexOptions=Index vector (dialog),Index vector (dialog)  Indices=1,2  OutputSizes=1,1
  Selector4 : Selector  NumberOfDimensions=2  InputPortWidth=3  IndexOptions=Index vector (dialog),Index vector (dialog)  Indices=2,1  OutputSizes=1,1
  Selector5 : Selector  NumberOfDimensions=2  InputPortWidth=3  IndexOptions=Index vector (dialog),Index vector (dialog)  Indices=2,3  OutputSizes=1,1
  Selector6 : Selector  NumberOfDimensions=2  InputPortWidth=3  IndexOptions=Index vector (dialog),Index vector (dialog)  Indices=3,2  OutputSizes=1,1
  Selector7 : Selector  NumberOfDimensions=2  InputPortWidth=3  IndexOptions=Index vector (dialog),Index vector (dialog)  Indices=3,1  OutputSizes=1,1
  Selector8 : Selector  NumberOfDimensions=2  InputPortWidth=3  IndexOptions=Index vector (dialog),Index vector (dialog)  Indices=1,3  OutputSizes=1,1
  Sum1 : Sum
  Sum2 : Sum
  Sum3 : Sum  Inputs=+-
  Vector Concatenate : Concatenate  NumInputs=4
  q_err : Outport
  wires:
  Divide1/1 -> Vector Concatenate/4
  Divide/1 -> Vector Concatenate/3
  Divide2/1 -> Vector Concatenate/1
  Sum2/1 -> Divide/1  "q3"
  Selector7/1 -> Sum3/1
  Selector5/1 -> Sum2/1
  Selector3/1 -> Sum1/1
  Selector8/1 -> Sum3/2
  Vector Concatenate/1 -> q_err/1
  A_I2B_err/1 -> Selector5/1, Selector6/1, Selector7/1, Selector8/1, Selector3/1, Selector4/1
  Gain9/1 -> Divide2/2, Divide/2, Divide1/2
  Sum1/1 -> Divide2/1  "q1"
  q2/1 -> Gain9/1, Vector Concatenate/2  "q2"
  Selector4/1 -> Sum1/2
  Sum3/1 -> Divide1/1  "q4"
  Selector6/1 -> Sum2/2

== system ADCS_orbiter_detumbling/Sensor and Attitude Determination/Subsystem3/Mapping choice/If Action Subsystem2/If Action Subsystem/If Action Subsystem ==
  q_err : Inport
  Action Port : ActionPort  ActionPortLabel=if(u1 == u2)
  q_err from q2 : Outport
  wires:
  q_err/1 -> q_err from q2/1

== system ADCS_orbiter_detumbling/Sensor and Attitude Determination/Subsystem3/Mapping choice/If Action Subsystem2/If Action Subsystem/If Action Subsystem1 ==
  A_I2B_err : Inport
  q3 : Inport  Port=2
  Action Port : ActionPort  ActionPortLabel=else
  From q3 : Subsystem
  q_err from q3 : Outport
  wires:
  From q3/1(q_err) -> q_err from q3/1
  A_I2B_err/1 -> From q3/1(A_I2B_err)
  q3/1 -> From q3/2(q3)

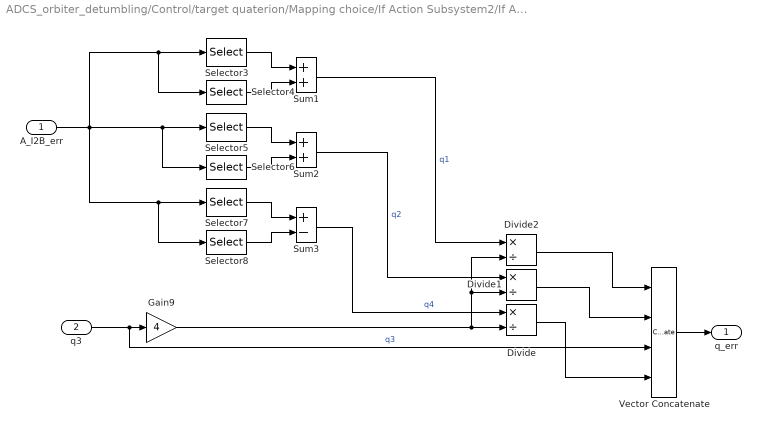
== system ADCS_orbiter_detumbling/Control/target quaterion/Mapping choice/If Action Subsystem2/If Action Subsystem/If Action Subsystem1/From q3 ==
  A_I2B_err : Inport
  q3 : Inport  Port=2
  Divide : Product  Inputs=*/
  Divide1 : Product  Inputs=*/
  Divide2 : Product  Inputs=*/
  Gain9 : Gain  Gain=4
  Selector3 : Selector  NumberOfDimensions=2  InputPortWidth=3  IndexOptions=Index vector (dialog),Index vector (dialog)  Indices=1,3  OutputSizes=1,1
  Selector4 : Selector  NumberOfDimensions=2  InputPortWidth=3  IndexOptions=Index vector (dialog),Index vector (dialog)  Indices=3,1  OutputSizes=1,1
  Selector5 : Selector  NumberOfDimensions=2  InputPortWidth=3  IndexOptions=Index vector (dialog),Index vector (dialog)  Indices=3,2  OutputSizes=1,1
  Selector6 : Selector  NumberOfDimensions=2  InputPortWidth=3  IndexOptions=Index vector (dialog),Index vector (dialog)  Indices=2,3  OutputSizes=1,1
  Selector7 : Selector  NumberOfDimensions=2  InputPortWidth=3  IndexOptions=Index vector (dialog),Index vector (dialog)  Indices=1,2  OutputSizes=1,1
  Selector8 : Selector  NumberOfDimensions=2  InputPortWidth=3  IndexOptions=Index vector (dialog),Index vector (dialog)  Indices=2,1  OutputSizes=1,1
  Sum1 : Sum
  Sum2 : Sum
  Sum3 : Sum  Inputs=+-
  Vector Concatenate : Concatenate  NumInputs=4
  q_err : Outport
  wires:
  Divide/1 -> Vector Concatenate/4
  Divide1/1 -> Vector Concatenate/2
  Divide2/1 -> Vector Concatenate/1
  Selector7/1 -> Sum3/1
  Selector5/1 -> Sum2/1
  Selector3/1 -> Sum1/1
  Selector8/1 -> Sum3/2
  Sum2/1 -> Divide1/1  "q2"
  Vector Concatenate/1 -> q_err/1
  A_I2B_err/1 -> Selector7/1, Selector8/1, Selector3/1, Selector4/1, Selector5/1, Selector6/1
  Gain9/1 -> Divide/2, Divide1/2, Divide2/2
  Sum1/1 -> Divide2/1  "q1"
  q3/1 -> Gain9/1, Vector Concatenate/3  "q3"
  Selector4/1 -> Sum1/2
  Sum3/1 -> Divide/1  "q4"
  Selector6/1 -> Sum2/2
